simulink model "slmips"  (R2015a)
settings: Solver=FixedStepDiscrete  StartTime=0.0  StopTime=20  FixedStep=1  RelTol=1e-3
libraries: simulink x43, hdlsllib x22
settings Model: PauseTimes=1  SnapshotInterval=1  LastModifiedBy=peselnikmg
settings DataIOCC: SaveOutput=off  SaveTime=off
settings OptimizationCC: BlockReduction=off  ConditionallyExecuteInputs=off  InlineParams=on  OptimizeModelRefInitCode=on  LifeSpan=1
settings DebuggingCC: AlgebraicLoopMsg=error
settings HardwareCC: ProdHWDeviceType=ASIC/FPGA->ASIC/FPGA  TargetLongLongMode=on  TargetIntDivRoundTo=Zero  TargetEndianess=LittleEndian  TargetHWDeviceType=MATLAB Host  ProdEqTarget=off
settings RTWCC: SystemTargetFile=ert.tlc  GenCodeOnly=on  TemplateMakefile=ert_default_tmf  Description=Embedded Coder  GenerateReport=on  IncludeHyperlinkInReport=on  LaunchReport=on  GenerateTraceInfo=on  GenerateTraceReport=on  GenerateTraceReportSl=on  GenerateTraceReportSf=on  GenerateTraceReportEml=on
settings CodeAppCC: IgnoreCustomStorageClasses=off
settings ERTTargetCC: ParMdlRefBuildCompliant=on  CompOptLevelCompliant=on  ConcurrentExecutionCompliant=on  ERTFirstTimeCompliant=on  SupportContinuousTime=off  SupportVariableSizeSignals=off  ModelStepFunctionPrototypeControlCompliant=on  CPPClassGenCompliant=on  InlinedParameterPlacement=Hierarchical  ERTCustomFileTemplate=example_file_process.tlc

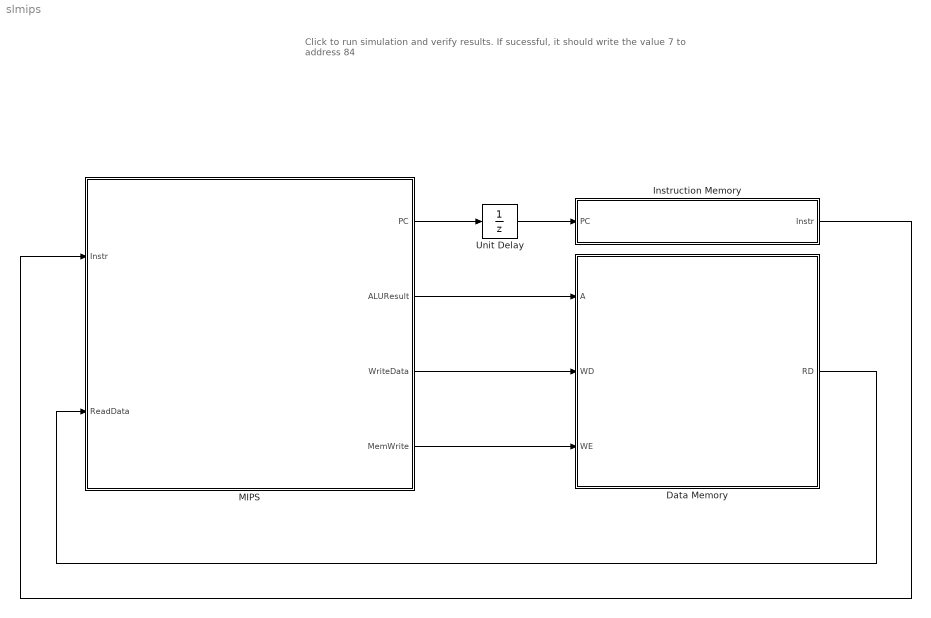
== system slmips ==
  note: Click to run simulation and verify results.
      | If sucessful, it should write the value 7 to address 84
  Data Memory : Subsystem
  Instruction Memory : Subsystem
  MIPS : Subsystem
  Unit Delay : UnitDelay  SampleTime=-1
  wires:
  MIPS/1(PC) -> Unit Delay/1
  Data Memory/1(RD) -> MIPS/2(ReadData)
  Instruction Memory/1(Instr) -> MIPS/1(Instr)
  Unit Delay/1 -> Instruction Memory/1(PC)
  MIPS/2(ALUResult) -> Data Memory/1(A)
  MIPS/3(WriteData) -> Data Memory/2(WD)
  MIPS/4(MemWrite) -> Data Memory/3(WE)

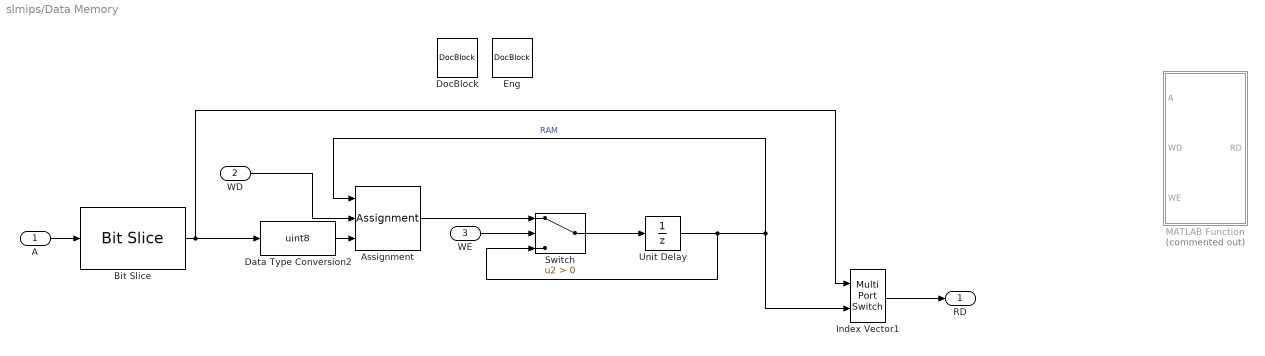
== system slmips/Data Memory ==
  A : Inport
  WD : Inport  Port=2
  WE : Inport  Port=3
  Assignment : Assignment  IndexMode=Zero-based  IndexOptions=Index vector (port)
  Bit Slice : hdlsllib/HDL Operations/Bit Slice  lidx=7  ridx=2
  Data Type Conversion2 : DataTypeConversion  OutDataTypeStr=uint8
  DocBlock : simulink/Model-Wide Utilities/DocBlock  DocumentType=Text
      content=|
      | Память данных имеет один порт чтения/записи. Если сигнал
      | разрешения записи WE равен единице, то данные со входа WD
      | записываются в ячейку памяти с адресом A по положительному фронту
      | тактового сигнала. Если же сигнал разрешения записи равен нулю,
      | то данные из ячейки с адресом A подаются на выход RD.
  Eng : simulink/Model-Wide Utilities/DocBlock  DocumentType=Text
      content=|
      | The data memory has a single read/write port. If the write enable,
      | WE, is 1, it writes data WD into address A on the rising edge of the clock.
      | If the write enable is 0, it reads address A onto RD.
  Index Vector1 : MultiPortSwitch  DataPortOrder=Zero-based contiguous  Inputs=1  zeroidx=on
  MATLAB Function : MATLAB Function  Commented=on  TreatAsAtomicUnit=on
  Switch : Switch  Criteria=u2 > Threshold
  Unit Delay : UnitDelay  InitialCondition=zeros(64,1)  SampleTime=-1
  RD : Outport  OutDataTypeStr=fixdt(0,32,0)
  wires:
  Unit Delay/1 -> Index Vector1/2, Assignment/1, Switch/3  "RAM"
  WE/1 -> Switch/2
  WD/1 -> Assignment/2
  Assignment/1 -> Switch/1
  Switch/1 -> Unit Delay/1
  Data Type Conversion2/1 -> Assignment/3
  Index Vector1/1 -> RD/1
  A/1 -> Bit Slice/1
  Bit Slice/1 -> Index Vector1/1, Data Type Conversion2/1

== system slmips/Instruction Memory ==
  PC : Inport
  DocBlock : simulink/Model-Wide Utilities/DocBlock  DocumentType=Text
      content=|
      | Память команд имеет один порт чтения. На адресный вход A подается
      | 32-битный адрес команды, после чего на выходе RD появляется
      | 32-битное число (т.е. команда), прочитанное из памяти по этому адресу.
  Eng : simulink/Model-Wide Utilities/DocBlock  DocumentType=Text
      content=|
      | The instruction memory has a single read port.1 It takes a 32-bit
      | instruction address input, A, and reads the 32-bit data (i.e., instruction)
      | from that address onto the read data output, RD.
  MATLAB Function : MATLAB Function  TreatAsAtomicUnit=on
  Instr : Outport  OutDataTypeStr=fixdt(0,32,0)
  wires:
  PC/1 -> MATLAB Function/1(PC)
  MATLAB Function/1(Instr) -> Instr/1  "Instr"

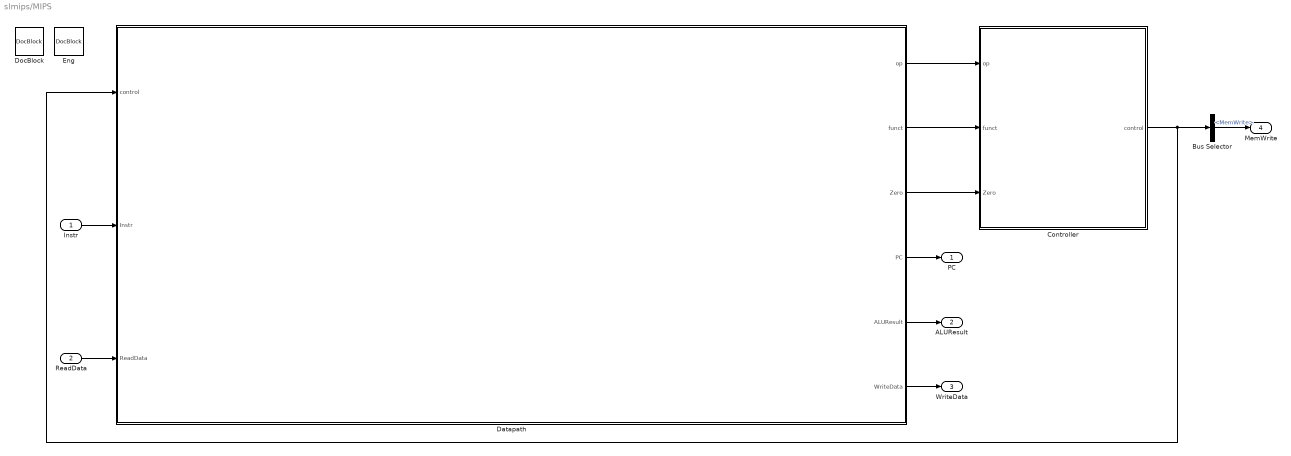
== system slmips/MIPS ==
  Instr : Inport
  ReadData : Inport  Port=2
  Bus Selector : BusSelector  OutputSignals=MemWrite
  Controller : Subsystem
  Datapath : Subsystem
  DocBlock : simulink/Model-Wide Utilities/DocBlock  DocumentType=Text
      content=|
      | Однотактовый процессор MIPS.
  Eng : simulink/Model-Wide Utilities/DocBlock  DocumentType=Text
      content=|
      | Single-cycle MIPS processor.
  PC : Outport
  ALUResult : Outport  Port=2
  WriteData : Outport  Port=3
  MemWrite : Outport  Port=4
  wires:
  Datapath/2(funct) -> Controller/2(funct)
  Datapath/1(op) -> Controller/1(op)
  Datapath/3(Zero) -> Controller/3(Zero)
  Datapath/4(PC) -> PC/1
  Instr/1 -> Datapath/2(Instr)
  ReadData/1 -> Datapath/3(ReadData)
  Datapath/6(WriteData) -> WriteData/1
  Datapath/5(ALUResult) -> ALUResult/1
  Bus Selector/1 -> MemWrite/1  "<MemWrite>"
  Controller/1(control) -> Datapath/1(control), Bus Selector/1

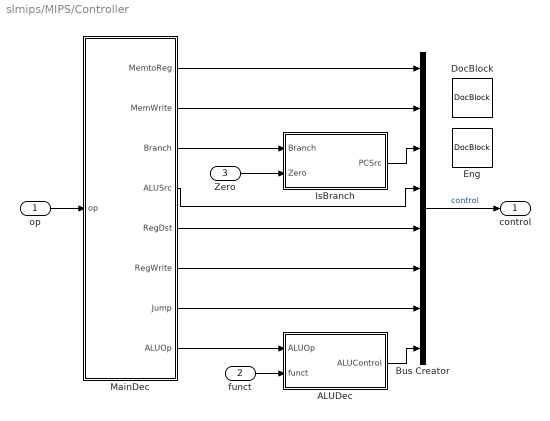
== system slmips/MIPS/Controller ==
  op : Inport
  funct : Inport  Port=2
  Zero : Inport  Port=3
  ALUDec : Subsystem
  Bus Creator : BusCreator  Inputs=8
  DocBlock : simulink/Model-Wide Utilities/DocBlock  DocumentType=Text
      content=|
      | Устройство управления формирует управляющие сигналы на основе
      | полей opcode и funct, присутствующих в каждой команде (Instr31:26 и
      | Instr5:0 соответственно).
  Eng : simulink/Model-Wide Utilities/DocBlock  DocumentType=Text
      content=|
      | The control unit computes the control signals based on the opcode and
      | funct fields of the instruction, Instr31:26 and Instr5:0.
  IsBranch : Subsystem
  MainDec : Subsystem
  control : Outport
  wires:
  Bus Creator/1 -> control/1  "control"
  MainDec/8(ALUOp) -> ALUDec/1(ALUOp)
  MainDec/3(Branch) -> IsBranch/1(Branch)
  op/1 -> MainDec/1(op)
  funct/1 -> ALUDec/2(funct)
  Zero/1 -> IsBranch/2(Zero)
  MainDec/1(MemtoReg) -> Bus Creator/1
  MainDec/2(MemWrite) -> Bus Creator/2
  IsBranch/1(PCSrc) -> Bus Creator/3
  MainDec/4(ALUSrc) -> Bus Creator/4
  MainDec/5(RegDst) -> Bus Creator/5
  MainDec/6(RegWrite) -> Bus Creator/6
  MainDec/7(Jump) -> Bus Creator/7
  ALUDec/1(ALUControl) -> Bus Creator/8

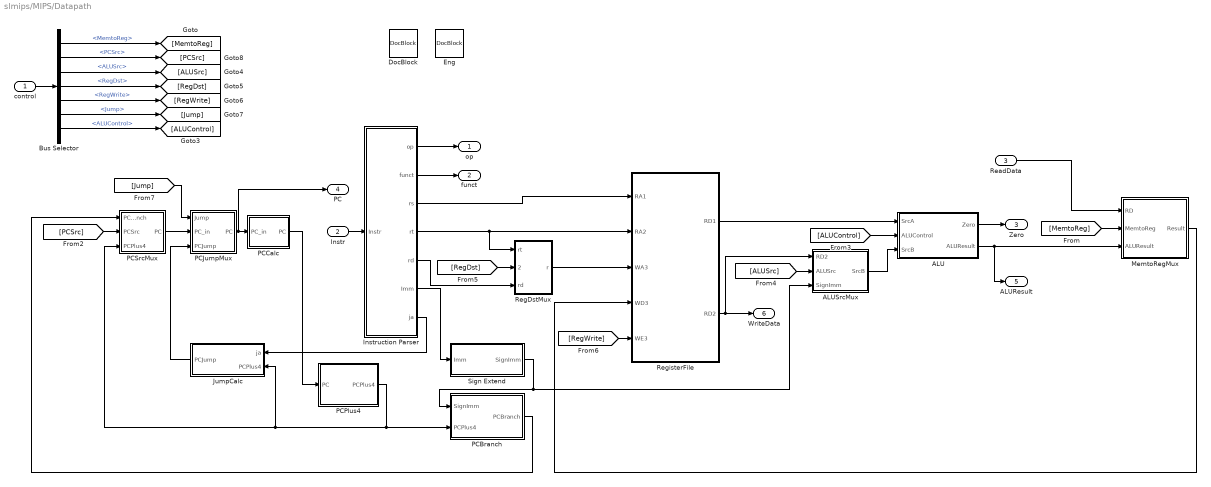
== system slmips/MIPS/Datapath ==
  control : Inport
  Instr : Inport  Port=2
  ReadData : Inport  Port=3
  ALU : Subsystem
  ALUSrcMux : Subsystem
  Bus Selector : BusSelector  OutputSignals=MemtoReg,PCSrc,ALUSrc,RegDst,RegWrite,Jump,ALUControl
  DocBlock : simulink/Model-Wide Utilities/DocBlock  DocumentType=Text
      content=|
      | Тракт данных однотактового процессора MIPS.
  Eng : simulink/Model-Wide Utilities/DocBlock  DocumentType=Text
      content=|
      | Datapath of a single-cycle MIPS processor.
  Instruction Parser : Subsystem
  JumpCalc : Subsystem
  MemtoRegMux : Subsystem
  PCBranch : Subsystem
  PCCalc : Subsystem
  PCJumpMux : Subsystem
  PCPlus4 : Subsystem
  PCSrcMux : Subsystem
  RegDstMux : Subsystem
  RegisterFile : Subsystem
  Sign Extend : Subsystem
  op : Outport
  funct : Outport  Port=2
  Zero : Outport  Port=3
  PC : Outport  Port=4
  ALUResult : Outport  Port=5
  WriteData : Outport  Port=6
  wires:
  Instruction Parser/4(rt) -> RegisterFile/2(RA2), RegDstMux/1(rt)
  [RegWrite] -> RegisterFile/5(WE3)
  Instruction Parser/3(rs) -> RegisterFile/1(RA1)
  ALUSrcMux/1(SrcB) -> ALU/3(SrcB)
  PCCalc/1(PC) -> PCPlus4/1(PC)
  [ALUSrc] -> ALUSrcMux/2(ALUSrc)
  RegisterFile/2(RD2) -> ALUSrcMux/1(RD2), WriteData/1
  [RegDst] -> RegDstMux/2(RegDst)
  [ALUControl] -> ALU/2(ALUControl)
  RegisterFile/1(RD1) -> ALU/1(SrcA)
  Sign Extend/1(SignImm) -> ALUSrcMux/3(SignImm), PCBranch/1(SignImm)
  RegDstMux/1(r) -> RegisterFile/3(WA3)
  [MemtoReg] -> MemtoRegMux/2(MemtoReg)
  Instr/1 -> Instruction Parser/1(Instr)
  Instruction Parser/2(funct) -> funct/1
  Instruction Parser/5(rd) -> RegDstMux/3(rd)
  Instruction Parser/6(Imm) -> Sign Extend/1(Imm)
  PCPlus4/1(PCPlus4) -> JumpCalc/2(PCPlus4), PCSrcMux/3(PCPlus4), PCBranch/2(PCPlus4)
  ALU/1(Zero) -> Zero/1
  PCBranch/1(PCBranch) -> PCSrcMux/1(PCBranch)
  Instruction Parser/1(op) -> op/1
  PCJumpMux/1(PC) -> PC/1, PCCalc/1(PC_in)
  [Jump] -> PCJumpMux/1(Jump)
  PCSrcMux/1(PC) -> PCJumpMux/2(PC_in)
  Instruction Parser/7(ja) -> JumpCalc/1(ja)
  JumpCalc/1(PCJump) -> PCJumpMux/3(PCJump)
  [PCSrc] -> PCSrcMux/2(PCSrc)
  control/1 -> Bus Selector/1
  Bus Selector/1 -> [MemtoReg]  "<MemtoReg>"
  Bus Selector/2 -> [PCSrc]  "<PCSrc>"
  Bus Selector/3 -> [ALUSrc]  "<ALUSrc>"
  Bus Selector/4 -> [RegDst]  "<RegDst>"
  Bus Selector/5 -> [RegWrite]  "<RegWrite>"
  Bus Selector/6 -> [Jump]  "<Jump>"
  Bus Selector/7 -> [ALUControl]  "<ALUControl>"
  ALU/2(ALUResult) -> MemtoRegMux/3(ALUResult), ALUResult/1
  ReadData/1 -> MemtoRegMux/1(RD)
  MemtoRegMux/1(Result) -> RegisterFile/4(WD3)

== system slmips/MIPS/Controller/ALUDec ==
  note: ALUOp
      | funct
      | ALUControl
      |
      | 00
      | X
      | 010 (addition)
      |
      | X1
      | X
      | 110 (subtraction)
      |
      | 1X
      | 100000
      | 010 (add)
      |
      | 1X
      | 100010
      | 110 (sub)
      |
      | 1X
      | 100100
      | 000 (and)
      |
      | 1X
      | 100101
      | 001 (or)
      |
      | 1X
      | 101010
      | 111 (slt)
  ALUOp : Inport
  funct : Inport  Port=2
  DocBlock : simulink/Model-Wide Utilities/DocBlock  DocumentType=Text
      content=|
      | Когда сигнал ALUOp равен 00 или 01, АЛУ должно складывать или
      | вычитать соответственно. Когда он равен 10, то значение ALUControl
      | должно определяться полем funct.
  Eng : simulink/Model-Wide Utilities/DocBlock  DocumentType=Text
      content=|
      | When ALUOp is 00 or 01,
      | the ALU should add or subtract, respectively. When ALUOp is 10, the
      | decoder examines the funct field to determine the ALUControl.
  MATLAB Function : MATLAB Function  TreatAsAtomicUnit=on
  ALUControl : Outport  OutDataTypeStr=fixdt(0,3,0)
  wires:
  ALUOp/1 -> MATLAB Function/1(ALUOp)
  funct/1 -> MATLAB Function/2(funct)
  MATLAB Function/1(ALUControl) -> ALUControl/1  "ALUControl"

== system slmips/MIPS/Controller/IsBranch ==
  Branch : Inport
  Zero : Inport  Port=2
  DocBlock : simulink/Model-Wide Utilities/DocBlock  DocumentType=Text
      content=|
      | Два регистра
      | сравниваются путем вычитания одного из другого в АЛУ. Если
      | ALUResult равен нулю, о чем сигнализирует флаг нуля, то регистры
      | равны. PCBranch
      | используется тогда, когда выполняется команда условного перехода и
      | установлен флаг нуля. Таким образом, сигнал Branch равен единице
      | для команды beq и нулю для прочих команд.
  Eng : simulink/Model-Wide Utilities/DocBlock  DocumentType=Text
      content=|
      | The two registers are compared by computing SrcA – SrcB using the
      | ALU. If ALUResult is 0, as indicated by the Zero flag from the ALU,
      | the registers are equal. We add a multiplexer to choose PC′ from either
      | PCPlus4 or PCBranch. PCBranch is selected if the instruction is a branch
      | and the Zero flag is asserted. Hence, Branch is 1 for beq and 0 for other
      | instructions.
  Logical Operator : Logic  AllPortsSameDT=off  OutDataTypeStr=fixdt(0,1,0)
  PCSrc : Outport
  wires:
  Zero/1 -> Logical Operator/2
  Logical Operator/1 -> PCSrc/1  "PCSrc"
  Branch/1 -> Logical Operator/1

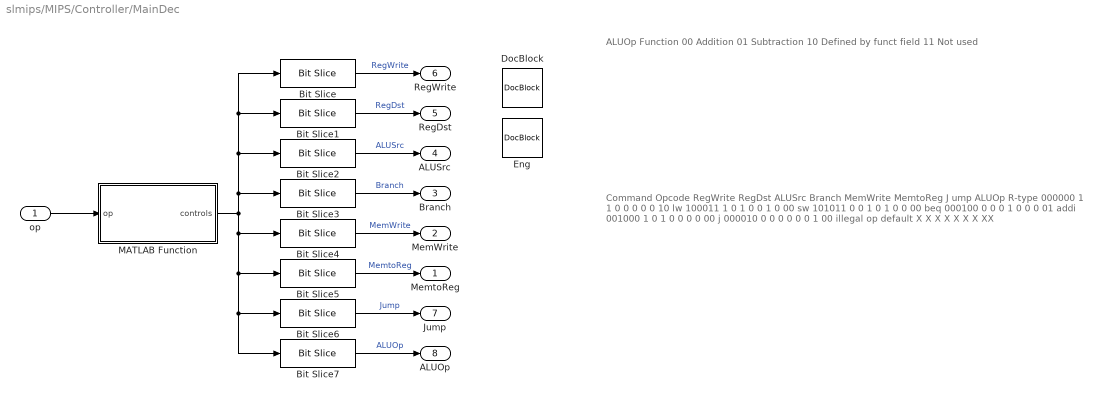
== system slmips/MIPS/Controller/MainDec ==
  note: Command
      | Opcode
      | RegWrite
      | RegDst
      | ALUSrc
      | Branch
      | MemWrite
      | MemtoReg
      | J ump
      | ALUOp
      |
      | R-type
      | 000000
      | 1
      | 1
      | 0
      | 0
      | 0
      | 0
      | 0
      | 10
      |
      | lw
      | 100011
      | 1
      | 0
      | 1
      | 0
      | 0
      | 1
      | 0
      | 00
      |
      | sw
      | 101011
      | 0
      | 0
      | 1
      | 0
      | 1
      | 0
      | 0
      | 00
      |
      | beq
      | 000100
      | 0
      | 0
      | 0
      | 1
      | 0
      | 0
      | 0
      | 01
      |
      | addi
      | 001000
      | 1
      | 0
      | 1
      | 0
      | 0
      | 0
      | 0
      | 00
      |
      | j
      | 000010
      | 0
      | 0
      | 0
      | 0
      | 0
      | 0
      | 1
      | 00
      |
      | illegal op
      | default
      | X
      | X
      | X
      | X
      | X
      | X
      | X
      | XX
  note: ALUOp
      | Function
      |
      | 00
      | Addition
      |
      | 01
      | Subtraction
      |
      | 10
      | Defined by funct field
      |
      | 11
      | Not used
  op : Inport
  Bit Slice : hdlsllib/HDL Operations/Bit Slice  lidx=8  ridx=8
  Bit Slice1 : hdlsllib/HDL Operations/Bit Slice  lidx=7  ridx=7
  Bit Slice2 : hdlsllib/HDL Operations/Bit Slice  lidx=6  ridx=6
  Bit Slice3 : hdlsllib/HDL Operations/Bit Slice  lidx=5  ridx=5
  Bit Slice4 : hdlsllib/HDL Operations/Bit Slice  lidx=4  ridx=4
  Bit Slice5 : hdlsllib/HDL Operations/Bit Slice  lidx=3  ridx=3
  Bit Slice6 : hdlsllib/HDL Operations/Bit Slice  lidx=2  ridx=2
  Bit Slice7 : hdlsllib/HDL Operations/Bit Slice  lidx=1  ridx=0
  DocBlock : simulink/Model-Wide Utilities/DocBlock  DocumentType=Text
      content=|
      | Основной дешифратор вычисляет значение большинства выходов на
      | основе поля opcode. Он также формирует двухбитный сигнал ALUOp.
      | Дешифратор АЛУ (ALU decoder) использует ALUOp совместно с полем
      | funct для вычисления состояния ALUControl. Расшифровка значений
      | сигнала ALUOp приведена в Таблице.
  Eng : simulink/Model-Wide Utilities/DocBlock  DocumentType=Text
      content=|
      | The main decoder
      | computes most of the outputs from the opcode. It also determines a 2-bit
      | ALUOp signal. The ALU decoder uses this ALUOp signal in conjunction
      | with the funct field to compute ALUControl. The meaning of the
      | ALUOp signal is given in Table.
  MATLAB Function : MATLAB Function  TreatAsAtomicUnit=on
  MemtoReg : Outport  OutDataTypeStr=fixdt(0,1,0)
  MemWrite : Outport  Port=2  OutDataTypeStr=fixdt(0,1,0)
  Branch : Outport  Port=3  OutDataTypeStr=fixdt(0,1,0)
  ALUSrc : Outport  Port=4  OutDataTypeStr=fixdt(0,1,0)
  RegDst : Outport  Port=5  OutDataTypeStr=fixdt(0,1,0)
  RegWrite : Outport  Port=6  OutDataTypeStr=fixdt(0,1,0)
  Jump : Outport  Port=7  OutDataTypeStr=fixdt(0,1,0)
  ALUOp : Outport  Port=8  OutDataTypeStr=fixdt(0,2,0)
  wires:
  op/1 -> MATLAB Function/1(op)
  MATLAB Function/1(controls) -> Bit Slice7/1, Bit Slice6/1, Bit Slice5/1, Bit Slice4/1, Bit Slice3/1, Bit Slice2/1, Bit Slice1/1, Bit Slice/1
  Bit Slice/1 -> RegWrite/1  "RegWrite"
  Bit Slice1/1 -> RegDst/1  "RegDst"
  Bit Slice2/1 -> ALUSrc/1  "ALUSrc"
  Bit Slice3/1 -> Branch/1  "Branch"
  Bit Slice4/1 -> MemWrite/1  "MemWrite"
  Bit Slice5/1 -> MemtoReg/1  "MemtoReg"
  Bit Slice6/1 -> Jump/1  "Jump"
  Bit Slice7/1 -> ALUOp/1  "ALUOp"

== system slmips/MIPS/Datapath/ALU ==
  note: ALUControl
      |
      | 010 (add)
      |
      | 110 (sub)
      |
      | 000 (and)
      |
      | 001 (or)
      |
      | 111 (slt)
  SrcA : Inport
  ALUControl : Inport  Port=2
  SrcB : Inport  Port=3
  DocBlock : simulink/Model-Wide Utilities/DocBlock  DocumentType=Text
      content=|
      | АЛУ получает на входы два операнда, SrcA и SrcB.
      | Трехбитный управляющий сигнал ALUControl
      | говорит АЛУ, какую операцию надо выполнить. На выходе из АЛУ
      | получается 32-битный результат ALUResult и флаг нуля (Zero flag),
      | который устанавливается в единицу, если ALUResult равен нулю.
  Eng : simulink/Model-Wide Utilities/DocBlock  DocumentType=Text
      content=|
      | The ALU receives two operands, SrcA and SrcB. SrcA
      | comes from the register file, and SrcB comes from the sign-extended
      | immediate. The 3-bit ALUControl signal specifies the operation. The
      | ALU generates a 32-bit ALUResult and a Zero flag, that indicates
      | whether ALUResult == 0.
  MATLAB Function : MATLAB Function  TreatAsAtomicUnit=on
  Zero : Outport  OutDataTypeStr=fixdt(0,1,0)
  ALUResult : Outport  Port=2  OutDataTypeStr=fixdt(0,32,0)
  wires:
  ALUControl/1 -> MATLAB Function/1(ALUControl)
  SrcA/1 -> MATLAB Function/2(SrcA)
  SrcB/1 -> MATLAB Function/3(SrcB)
  MATLAB Function/1(ALUResult) -> ALUResult/1
  MATLAB Function/2(Zero) -> Zero/1

== system slmips/MIPS/Datapath/ALUSrcMux ==
  RD2 : Inport
  ALUSrc : Inport  Port=2
  SignImm : Inport  Port=3
  ALUSrcMux : Switch  Criteria=u2 > Threshold
  DocBlock : simulink/Model-Wide Utilities/DocBlock  DocumentType=Text
      content=|
      | Нам пришлось добавить мультиплексор, чтобы была возможность
      | подать на вход АЛУ или SignImm, или выход RD2 регистрового файла.
      | Мультиплексор управляется новым сигналом ALUSrc.
      | ALUSrc равен нулю для команд типа R – в этом случае на вход АЛУ подается
      | значение из регистрового файла. Для команд lw и sw ALUSrc равен
      | единице, и на вход АЛУ подается SignImm.
  Eng : simulink/Model-Wide Utilities/DocBlock  DocumentType=Text
      content=|
      | The multiplexer to choose SrcB from either the register file RD2 port
      | or SignImm.
      | The multiplexer is controlled by a new signal, ALUSrc. ALUSrc is 0
      | for R-type instructions to choose SrcB from the register file; it is 1 for
      | lw and sw to choose SignImm. This principle of enhancing the datapath’s
      | capabilities by adding a multiplexer to choose inputs from several possibilities
      | is extremely useful. Indeed, we will apply it twice more to complete
      | the handling of R-type instructions.
  SrcB : Outport
  wires:
  ALUSrc/1 -> ALUSrcMux/2
  ALUSrcMux/1 -> SrcB/1
  SignImm/1 -> ALUSrcMux/1
  RD2/1 -> ALUSrcMux/3

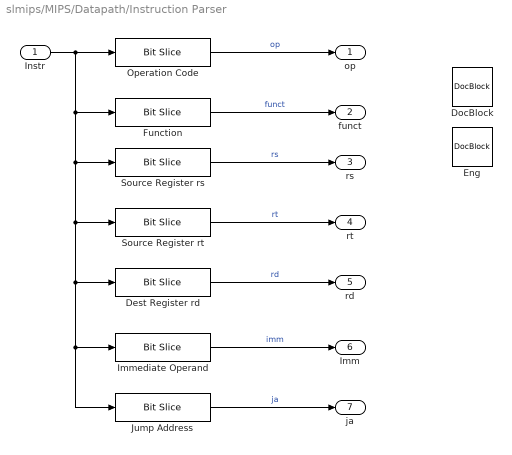
== system slmips/MIPS/Datapath/Instruction Parser ==
  Instr : Inport
  Dest Register rd : hdlsllib/HDL Operations/Bit Slice  lidx=15  ridx=11
  DocBlock : simulink/Model-Wide Utilities/DocBlock  DocumentType=Text
      content=|
      | Refer to MIPS machine code description.
  Eng : simulink/Model-Wide Utilities/DocBlock  DocumentType=Text
      content=|
      | Refer to MIPS machine code description.
  Function : hdlsllib/HDL Operations/Bit Slice  lidx=5  ridx=0
  Immediate Operand : hdlsllib/HDL Operations/Bit Slice  lidx=15  ridx=0
  Jump Address : hdlsllib/HDL Operations/Bit Slice  lidx=25  ridx=0
  Operation Code : hdlsllib/HDL Operations/Bit Slice  lidx=31  ridx=26
  Source Register rs : hdlsllib/HDL Operations/Bit Slice  lidx=25  ridx=21
  Source Register rt : hdlsllib/HDL Operations/Bit Slice  lidx=20  ridx=16
  op : Outport
  funct : Outport  Port=2
  rs : Outport  Port=3
  rt : Outport  Port=4
  rd : Outport  Port=5
  Imm : Outport  Port=6
  ja : Outport  Port=7
  wires:
  Source Register rs/1 -> rs/1  "rs"
  Immediate Operand/1 -> Imm/1  "imm"
  Source Register rt/1 -> rt/1  "rt"
  Dest Register rd/1 -> rd/1  "rd"
  Instr/1 -> Operation Code/1, Function/1, Jump Address/1, Immediate Operand/1, Dest Register rd/1, Source Register rt/1, Source Register rs/1
  Operation Code/1 -> op/1  "op"
  Function/1 -> funct/1  "funct"
  Jump Address/1 -> ja/1  "ja"

== system slmips/MIPS/Datapath/JumpCalc ==
  note: Do we need this? From diagram on p. 960, seems yes.. But logically - no!
  ja : Inport
  PCPlus4 : Inport  Port=2
  Bit Concat : hdlsllib/HDL Operations/Bit Concat  numInputs=3
  Bit Shift : hdlsllib/HDL Operations/Bit Shift  Commented=through  mode=Shift Left Logical  N=2
  Constant : Constant  Value=0  OutDataTypeStr=fixdt(0,2,0)
  DocBlock : simulink/Model-Wide Utilities/DocBlock  DocumentType=Text
      content=|
      | Команда безусловного перехода j записывает новое значение в счетчик команд.
      | Два младших бита нового значения всегда равны нулю, потому что длина любой
      | команды равна четырем байтам, следовательно, ее адрес всегда кратен
      | четырем. Следующие 26 бит процессор возьмет из поля адреса перехода (jump
      | address field) Instr25:0. Четыре оставшихся старших бита будут равны четырем
      | старшим битам предыдущего значения счетчика команд.
  Eng : simulink/Model-Wide Utilities/DocBlock  DocumentType=Text
      content=|
      | The jump instruction, j, writes a new value into the PC. The two least significant
      | bits of the PC are always 0, because the PC is word aligned (i.e., always a multiple
      | of 4). The next 26 bits are taken from the jump address field in Instr25:0. The
      | upper four bits are taken from the old value of the PC.
  Operation Code : hdlsllib/HDL Operations/Bit Slice  lidx=31  ridx=28
  PCJump : Outport
  wires:
  Bit Concat/1 -> PCJump/1
  PCPlus4/1 -> Operation Code/1
  ja/1 -> Bit Concat/2
  Operation Code/1 -> Bit Concat/1
  Constant/1 -> Bit Concat/3

== system slmips/MIPS/Datapath/MemtoRegMux ==
  RD : Inport
  MemtoReg : Inport  Port=2
  ALUResult : Inport  Port=3
  DocBlock : simulink/Model-Wide Utilities/DocBlock  DocumentType=Text
      content=|
      | Команды типа R должны записывать в
      | регистровый файл значение ALUResult. Чтобы выбирать между
      | ReadData и ALUResult, мы добавляем этот мультиплексор.
      | Этот мультиплексор управляется сигналом MemtoReg.
      | MemtoReg равен нулю для команд
      | типа R – в этом случае Result принимает значение ALUResult.
      | Для команды lw MemtoReg равен единице, а Result принимает
      | значение ReadData. Для команды sw значение MemtoReg не играет
      | никакой роли, так как sw ничего в регистровый файл не пишет.
  Eng : simulink/Model-Wide Utilities/DocBlock  DocumentType=Text
      content=|
      | R-type instructions write the ALUResult to the register
      | file. Therefore, we add this multiplexer to choose between ReadData
      | and ALUResult. We call its output Result. This multiplexer is
      | controlled by signal MemtoReg. MemtoReg is 0 for R-type
      | instructions to choose Result from the ALUResult; it is 1 for lw to choose
      | ReadData. We don’t care about the value of MemtoReg for sw, because
      | sw does not write to the register file.
  MemtoRegMux : Switch  Criteria=u2 > Threshold
  Result : Outport
  wires:
  MemtoReg/1 -> MemtoRegMux/2
  MemtoRegMux/1 -> Result/1
  RD/1 -> MemtoRegMux/1
  ALUResult/1 -> MemtoRegMux/3

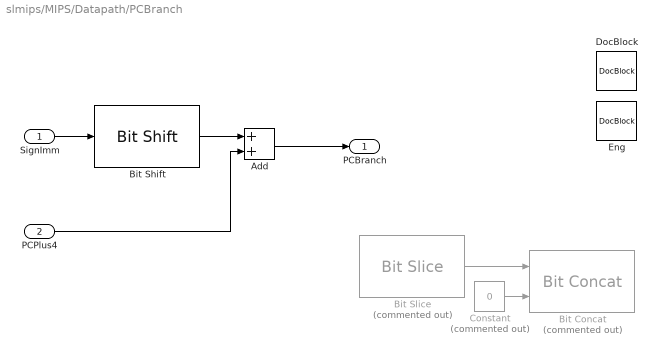
== system slmips/MIPS/Datapath/PCBranch ==
  SignImm : Inport
  PCPlus4 : Inport  Port=2
  Add : Sum  AccumDataTypeStr=fixdt(0,32,0)  OutDataTypeStr=fixdt(0,32,0)
  Bit Concat : hdlsllib/HDL Operations/Bit Concat  Commented=on  numInputs=2
  Bit Shift : hdlsllib/HDL Operations/Bit Shift  mode=Shift Left Logical  N=2
  Bit Slice : hdlsllib/HDL Operations/Bit Slice  Commented=on  lidx=29  ridx=0
  Constant : Constant  Commented=on  Value=0  OutDataTypeStr=fixdt(0,2,0)
  DocBlock : simulink/Model-Wide Utilities/DocBlock  DocumentType=Text
      content=|
      | Смещение указывает, сколько команд нужно перепрыгнуть, прежде чем
      | продолжить выполнение программы. Таким образом, над значением
      | непосредственного операнда надо выполнить операцию знакового
      | расширения, поле чего умножить его на четыре, чтобы получить новое
      | значение счетчика команд: PC_in = PC + 4 + SignImm * 4.
      | Новое значение счетчика команд на случай выполненного
      | условного перехода (PCBranch) вычисляется путем сдвига SignImm
      | влево на два разряда и последующего сложения с PCPlus4.
  Eng : simulink/Model-Wide Utilities/DocBlock  DocumentType=Text
      content=|
      | The offset
      | indicates the number of instructions to branch past. Hence, the immediate
      | must be sign-extended and multiplied by 4 to get the new program counter
      | value: PC′ = PC + 4 + SignImm × 4.
      | The next PC value
      | for a taken branch, PCBranch, is computed by shifting SignImm left
      | by 2 bits, then adding it to PCPlus4.
  PCBranch : Outport
  wires:
  SignImm/1 -> Bit Shift/1
  PCPlus4/1 -> Add/2
  Bit Shift/1 -> Add/1
  Add/1 -> PCBranch/1
  Bit Slice/1 -> Bit Concat/1
  Constant/1 -> Bit Concat/2

== system slmips/MIPS/Datapath/PCCalc ==
  PC_in : Inport
  DocBlock : simulink/Model-Wide Utilities/DocBlock  DocumentType=Text
      content=|
      | Счетчик команд – это обычный 32-битный регистр. Его выход (PC)
      | содержит адрес текущей команды. Его вход (PC_in) содержит адрес
      | следующей команды.
  Eng : simulink/Model-Wide Utilities/DocBlock  DocumentType=Text
      content=|
      | The program counter is an ordinary 32-bit register. Its output, PC,
      | points to the current instruction. Its input, PC′, indicates the address of
      | the next instruction.
  PC Start : UnitDelay  Description=Начальное значение счетчика команд.  SampleTime=-1
  PC : Outport  OutDataTypeStr=fixdt(0,32,0)
  wires:
  PC_in/1 -> PC Start/1
  PC Start/1 -> PC/1  "PC"

== system slmips/MIPS/Datapath/PCJumpMux ==
  Jump : Inport
  PC_in : Inport  Port=2
  PCJump : Inport  Port=3
  DocBlock : simulink/Model-Wide Utilities/DocBlock  DocumentType=Text
      content=|
      | Команда безусловного перехода j записывает новое значение в счетчик команд.
      | Два младших бита нового значения всегда равны нулю, потому что длина любой
      | команды равна четырем байтам, следовательно, ее адрес всегда кратен
      | четырем. Следующие 26 бит процессор возьмет из поля адреса перехода (jump
      | address field) Instr25:0. Четыре оставшихся старших бита будут равны четырем
      | старшим битам предыдущего значения счетчика команд.
  Eng : simulink/Model-Wide Utilities/DocBlock  DocumentType=Text
      content=|
      | The jump instruction, j, writes a new value into the PC. The two least significant
      | bits of the PC are always 0, because the PC is word aligned (i.e., always a multiple
      | of 4). The next 26 bits are taken from the jump address field in Instr25:0. The
      | upper four bits are taken from the old value of the PC.
  PCJumpMux : Switch  Criteria=u2 > Threshold
  PC : Outport
  wires:
  PCJumpMux/1 -> PC/1
  Jump/1 -> PCJumpMux/2
  PCJump/1 -> PCJumpMux/1
  PC_in/1 -> PCJumpMux/3

== system slmips/MIPS/Datapath/PCPlus4 ==
  PC : Inport
  DocBlock : simulink/Model-Wide Utilities/DocBlock  DocumentType=Text
      content=|
      | Одновременно с выполнением команды процессор должен вычислить
      | адрес следующей команды, PC_in. Так как команды 32-битные, то есть
      | четырехбайтные, то адрес следующей команды равен PC + 4.
  Eng : simulink/Model-Wide Utilities/DocBlock  DocumentType=Text
      content=|
      | While the instruction is being executed, the processor must compute the
      | address of the next instruction, PC′. Because instructions are 32 bits =
      | 4 bytes, the next instruction is at PC + 4.
  PCInc : Bias  Bias=4
  PCPlus4 : Outport
  wires:
  PC/1 -> PCInc/1
  PCInc/1 -> PCPlus4/1

== system slmips/MIPS/Datapath/PCSrcMux ==
  PCBranch : Inport
  PCSrc : Inport  Port=2
  PCPlus4 : Inport  Port=3
  DocBlock : simulink/Model-Wide Utilities/DocBlock  DocumentType=Text
      content=|
      | Мультиплексор, чтобы выбрать, какое именно
      | значение присвоить PC_in – PCPlus4 или PCBranch. PCBranch
      | используется тогда, когда выполняется команда условного перехода и
      | установлен флаг нуля.
  Eng : simulink/Model-Wide Utilities/DocBlock  DocumentType=Text
      content=|
      | The multiplexer to choose PC′ from either
      | PCPlus4 or PCBranch. PCBranch is selected if the instruction is a branch
      | and the Zero flag is asserted.
  PCSrcMux : Switch  Criteria=u2 > Threshold
  PC : Outport
  wires:
  PCSrc/1 -> PCSrcMux/2
  PCPlus4/1 -> PCSrcMux/3
  PCSrcMux/1 -> PC/1
  PCBranch/1 -> PCSrcMux/1

== system slmips/MIPS/Datapath/RegDstMux ==
  rt : Inport
  RegDst : Inport  Port=2
  rd : Inport  Port=3
  DocBlock : simulink/Model-Wide Utilities/DocBlock  DocumentType=Text
      content=|
      | Этот мультиплексор
      | управляется сигналом RegDst. RegDst равен единице для команд
      | типа R – в этом случае выход принимает значение поля rd (Instr15:11).
      | Для команды lw RegDst равен нулю, а выход принимает значение
      | поля rt (Instr20:16). Для команды sw значение RegDst не играет никакой
      | роли, так как sw ничего в регистровый файл не пишет.
  Eng : simulink/Model-Wide Utilities/DocBlock  DocumentType=Text
      content=|
      | The multiplexer is controlled by RegDst. RegDst is 1 for R-type
      | instructions to choose WriteReg from the rd field, Instr15:11; it is 0 for
      | lw to choose the rt field, Instr20:16. We don’t care about the value of
      | RegDst for sw, because sw does not write to the register file.
  RegDstMux : Switch  Criteria=u2 > Threshold
  r : Outport
  wires:
  RegDst/1 -> RegDstMux/2
  RegDstMux/1 -> r/1
  rt/1 -> RegDstMux/3
  rd/1 -> RegDstMux/1

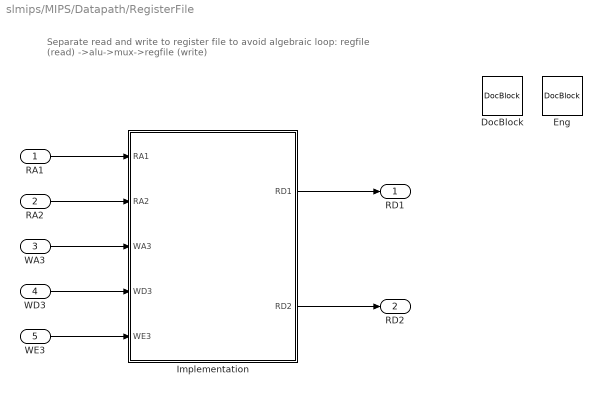
== system slmips/MIPS/Datapath/RegisterFile ==
  note: Separate read and write to register file to avoid algebraic loop:
      | regfile (read) ->alu->mux->regfile (write)
  RA1 : Inport
  RA2 : Inport  Port=2
  WA3 : Inport  Port=3
  WD3 : Inport  Port=4
  WE3 : Inport  Port=5
  DocBlock : simulink/Model-Wide Utilities/DocBlock  DocumentType=Text
      content=|
      | Регистровый файл, содержащий 32 элемента по 32 бита каждый, имеет
      | два порта чтения и один порт записи данных. Порты чтения имеют
      | пятибитные входы адреса A1 и A2, каждый из которых определяет один
      | из 2^5 = 32 регистров в качестве источника данных для команды. Каждый
      | из портов читает 32-битное значение из регистра и подает его на
      | выходы RD1 и RD2 соответственно. Порт записи получает пятибитный
      | адрес регистра на адресный вход A3, 32-битное число на вход данных
      | WD, сигнал разрешения записи WE3 и тактовый сигнал. Если сигнал
      | разрешения записи равен единице, то регистровый файл записывает
      | данные в указанный регистр по положительному фронту тактового
      | сигнала.
  Eng : simulink/Model-Wide Utilities/DocBlock  DocumentType=Text
      content=|
      | The 32-element × 32-bit register file has two read ports and one write
      | port. The read ports take 5-bit address inputs, A1 and A2, each specifying
      | one of 25 = 32 registers as source operands. They read the 32-bit register
      | values onto read data outputs RD1 and RD2, respectively. The write port
      | takes a 5-bit address input, A3; a 32-bit write data input, WD; a write
      | enable input, WE3; and a clock. If the write enable is 1, the register file
      | writes the data into the specified register on the rising edge of the clock.
  Implementation : Subsystem  Variant=on  OverrideUsingVariant=SL_impl_BB
  RD1 : Outport  OutDataTypeStr=fixdt(0,32,0)
  RD2 : Outport  Port=2  OutDataTypeStr=fixdt(0,32,0)
  wires:
  RA1/1 -> Implementation/1(RA1)
  RA2/1 -> Implementation/2(RA2)
  WA3/1 -> Implementation/3(WA3)
  WD3/1 -> Implementation/4(WD3)
  WE3/1 -> Implementation/5(WE3)
  Implementation/1(RD1) -> RD1/1
  Implementation/2(RD2) -> RD2/1

== system slmips/MIPS/Datapath/Sign Extend ==
  note: TODO: check if it works with jumping back. PCBranch must decrement in this case.
  Imm : Inport
  Data Type Conversion : DataTypeConversion  Commented=on  ConvertRealWorld=Stored Integer (SI)
  DocBlock : simulink/Model-Wide Utilities/DocBlock  DocumentType=Text
      content=|
      | Команде lw также требуется смещение (offset) – число, которое будет
      | прибавлено к базовому адресу. Смещение передается как
      | непосредственный операнд (immediate), то есть находится
      | непосредственно в поле Instr15:0, занимая младшие 16 бит. Так как
      | 16-битное число может быть как положительным, так и отрицательным,
      | то над ним должна быть выполнена операция знакового расширения до
      | 32 бит. Полученное 32-битное расширенное значение называется SignImm.
      | Знаковое расширение заключается в том, что знаковый бит (он же
      | старший бит) расширяемого числа просто копируется во все старшие
      | биты расширенного числа, а именно SignImm15:0 = Instr15:0 и
      | SignImm31:16 = Instr15.
  Eng : simulink/Model-Wide Utilities/DocBlock  DocumentType=Text
      content=|
      | The lw instruction also requires an offset. The offset is stored in the
      | immediate field of the instruction, Instr15:0. Because the 16-bit immediate
      | might be either positive or negative, it must be sign-extended to 32 bits.
      | The 32-bit sign-extended value is called SignImm.
      | Sign extension simply copies the sign bit
      | (most significant bit) of a short input into all of the upper bits of the
      | longer output. Specifically, SignImm15:0 = Instr15:0 and SignImm31:16 =
      | Instr15.
  MATLAB Function : MATLAB Function  TreatAsAtomicUnit=on
  SignImm : Outport  OutDataTypeStr=fixdt(0,32,0)
  wires:
  Imm/1 -> MATLAB Function/1(a)
  MATLAB Function/1(y) -> SignImm/1

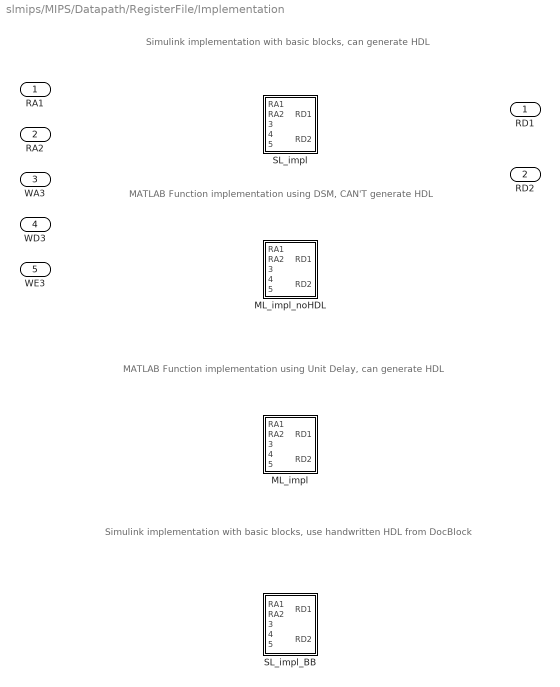
== system slmips/MIPS/Datapath/RegisterFile/Implementation ==
  note: MATLAB Function implementation using DSM, CAN'T generate HDL
  note: Simulink implementation with basic blocks, can generate HDL
  note: MATLAB Function implementation using Unit Delay, can generate HDL
  note: Simulink implementation with basic blocks, use handwritten HDL from DocBlock
  RA1 : Inport
  RA2 : Inport  Port=2
  WA3 : Inport  Port=3
  WD3 : Inport  Port=4
  WE3 : Inport  Port=5
  ML_impl : Subsystem  VariantControl=ML_impl
  ML_impl_noHDL : Subsystem  VariantControl=ML_impl_noHDL
  SL_impl : Subsystem  VariantControl=SL_impl
  SL_impl_BB : Subsystem  VariantControl=SL_impl_BB
  RD1 : Outport  OutDataTypeStr=fixdt(0,32,0)
  RD2 : Outport  Port=2  OutDataTypeStr=fixdt(0,32,0)

== system slmips/MIPS/Datapath/RegisterFile/Implementation/ML_impl ==
  RA1 : Inport
  RA2 : Inport  Port=2
  WA3 : Inport  Port=3
  WD3 : Inport  Port=4
  WE3 : Inport  Port=5
  Read : MATLAB Function  TreatAsAtomicUnit=on
  Unit Delay : UnitDelay  InitialCondition=zeros(32,1)  SampleTime=-1
  Write : MATLAB Function  TreatAsAtomicUnit=on
  RD1 : Outport  OutDataTypeStr=fixdt(0,32,0)
  RD2 : Outport  Port=2  OutDataTypeStr=fixdt(0,32,0)
  wires:
  WD3/1 -> Write/2(WD3)
  RA1/1 -> Read/1(RA1)
  RA2/1 -> Read/2(RA2)
  WA3/1 -> Write/1(WA3)
  WE3/1 -> Write/3(WE3)
  Read/2(RD2) -> RD2/1
  Read/1(RD1) -> RD1/1
  Write/1(regfile_wr) -> Unit Delay/1
  Unit Delay/1 -> Write/4(regfile), Read/3(regfile)

== system slmips/MIPS/Datapath/RegisterFile/Implementation/ML_impl_noHDL ==
  RA1 : Inport
  RA2 : Inport  Port=2
  WA3 : Inport  Port=3
  WD3 : Inport  Port=4
  WE3 : Inport  Port=5
  Data Store Memory : DataStoreMemory  DataStoreName=regfile  WriteAfterWriteMsg=warning  InitialValue=zeros(32,1)  OutDataTypeStr=fixdt(0,32,0)
  Read : MATLAB Function  TreatAsAtomicUnit=on
  Write : MATLAB Function  TreatAsAtomicUnit=on
  RD1 : Outport  OutDataTypeStr=fixdt(0,32,0)
  RD2 : Outport  Port=2  OutDataTypeStr=fixdt(0,32,0)
  wires:
  Read/1(RD1) -> RD1/1
  Read/2(RD2) -> RD2/1
  WE3/1 -> Write/3(WE3)
  WA3/1 -> Write/1(WA3)
  RA2/1 -> Read/2(RA2)
  RA1/1 -> Read/1(RA1)
  WD3/1 -> Write/2(WD3)

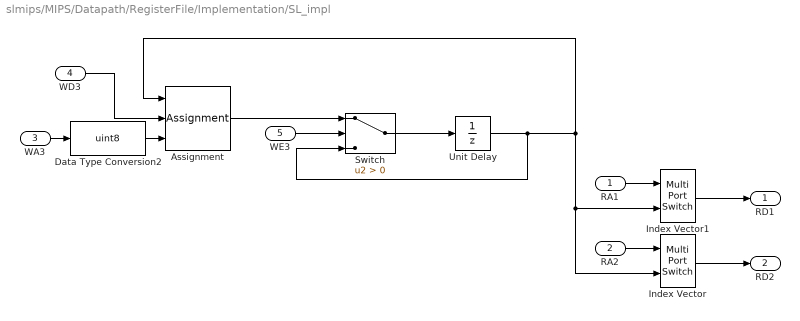
== system slmips/MIPS/Datapath/RegisterFile/Implementation/SL_impl ==
  RA1 : Inport
  RA2 : Inport  Port=2
  WA3 : Inport  Port=3
  WD3 : Inport  Port=4
  WE3 : Inport  Port=5
  Assignment : Assignment  IndexMode=Zero-based  IndexOptions=Index vector (port)
  Data Type Conversion2 : DataTypeConversion  OutDataTypeStr=uint8
  Index Vector : MultiPortSwitch  DataPortOrder=Zero-based contiguous  Inputs=1  zeroidx=on
  Index Vector1 : MultiPortSwitch  DataPortOrder=Zero-based contiguous  Inputs=1  zeroidx=on
  Switch : Switch  Criteria=u2 > Threshold
  Unit Delay : UnitDelay  InitialCondition=zeros(32,1)  SampleTime=-1
  RD1 : Outport  OutDataTypeStr=fixdt(0,32,0)
  RD2 : Outport  Port=2  OutDataTypeStr=fixdt(0,32,0)
  wires:
  Unit Delay/1 -> Index Vector1/2, Index Vector/2, Assignment/1, Switch/3
  Index Vector/1 -> RD2/1
  RA2/1 -> Index Vector/1
  WE3/1 -> Switch/2
  WA3/1 -> Data Type Conversion2/1
  WD3/1 -> Assignment/2
  Assignment/1 -> Switch/1
  Switch/1 -> Unit Delay/1
  Data Type Conversion2/1 -> Assignment/3
  RA1/1 -> Index Vector1/1
  Index Vector1/1 -> RD1/1

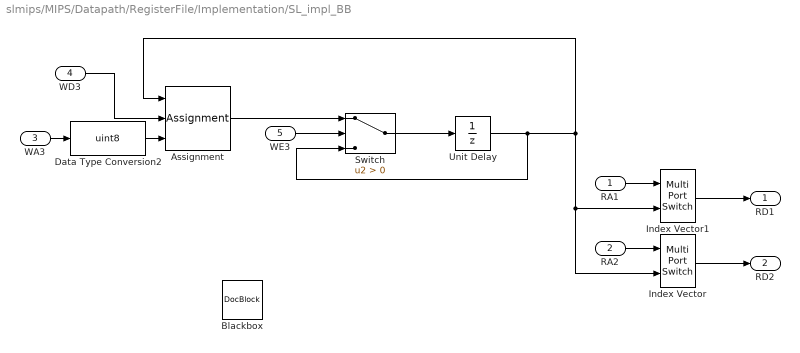
== system slmips/MIPS/Datapath/RegisterFile/Implementation/SL_impl_BB ==
  RA1 : Inport
  RA2 : Inport  Port=2
  WA3 : Inport  Port=3
  WD3 : Inport  Port=4
  WE3 : Inport  Port=5
  Assignment : Assignment  IndexMode=Zero-based  IndexOptions=Index vector (port)
  Blackbox : simulink/Model-Wide Utilities/DocBlock  DocumentType=Text
      content=|
      | module SL_impl_BB(
      |            clk,
      |            RA1,
      |            RA2,
      |            WA3,
      |            WD3,
      |            WE3,
      |            RD1,
      |            RD2
      |           );
      |
      | input   clk;
      | input   [4:0] RA1;  // ufix5
      | input   [4:0] RA2;  // ufix5
      | input   [4:0] WA3;  // ufix5
      | input   [31:0] WD3;  // uint32
      | input   WE3;  // ufix1
      | output  [31:0] RD1;  // uint32
      | output  [31:0] RD2;  // uint32
      |
      | reg [31:0] rf[31:0];
      |
      | always @(posedge clk)
      |     if (WE3) rf[WA3] <= WD3;
      |
      | assign RD1 = (RA1 != 0) ? rf[RA1] : 0;
      | assign RD2 = (RA2 != 0) ? rf[RA2] : 0;
      |
      | endmodule
  Data Type Conversion2 : DataTypeConversion  OutDataTypeStr=uint8
  Index Vector : MultiPortSwitch  DataPortOrder=Zero-based contiguous  Inputs=1  zeroidx=on
  Index Vector1 : MultiPortSwitch  DataPortOrder=Zero-based contiguous  Inputs=1  zeroidx=on
  Switch : Switch  Criteria=u2 > Threshold
  Unit Delay : UnitDelay  InitialCondition=zeros(32,1)  SampleTime=-1
  RD1 : Outport  OutDataTypeStr=fixdt(0,32,0)
  RD2 : Outport  Port=2  OutDataTypeStr=fixdt(0,32,0)
  wires:
  Unit Delay/1 -> Index Vector1/2, Index Vector/2, Assignment/1, Switch/3
  Index Vector/1 -> RD2/1
  RA2/1 -> Index Vector/1
  WE3/1 -> Switch/2
  WA3/1 -> Data Type Conversion2/1
  WD3/1 -> Assignment/2
  Assignment/1 -> Switch/1
  Switch/1 -> Unit Delay/1
  Data Type Conversion2/1 -> Assignment/3
  RA1/1 -> Index Vector1/1
  Index Vector1/1 -> RD1/1

== matlab function slmips/MIPS/Datapath/ALU/MATLAB Function ==
  settings: fimath=|
      | fimath(...
      | 'RoundMode', 'floor',...
      | 'OverflowMode', 'wrap',...
      | 'ProductMode', 'FullPrecision', 'ProductWordLength', 32,...
      | 'SumMode', 'FullPrecision', 'SumWordLength', 32,...
      | 'CastBeforeSum', true);
  data: ALUControl input fixdt(0,3,0); ALUResult output fixdt(0,32,0); SrcA input fixdt(0,32,0); SrcB input fixdt(0,32,0); Zero output fixdt(0,1,0)
function [ALUResult, Zero] = fcn(ALUControl, SrcA, SrcB)
%#codegen

ALUResult = fi(0,0,32,0);
Zero = fi(0,0,1,0);

switch ALUControl
    case bin2dec('010')
        %add
        ALUResult(:) = SrcA + SrcB;
    case bin2dec('110')
        %sub
        ALUResult(:) = SrcA - SrcB;
    case bin2dec('000')
        %and
        ALUResult(:) = bitand(SrcA, SrcB);
    case bin2dec('001')
        %or
        ALUResult(:) = bitor(SrcA, SrcB);
    case bin2dec('111')
        %slt
        if (SrcA < SrcB)
            ALUResult(:) = 1;
        else
            ALUResult(:) = 0;
        end
    otherwise
end

%slt
if (ALUResult == 0)
    Zero(:) = 1;
else
    Zero(:) = 0;
end

== matlab function slmips/MIPS/Datapath/Sign Extend/MATLAB Function ==
  data: a input fixdt(0,16,0); y output fixdt(0,32,0)
function y = fcn(a)
%#codegen

%Output is a signed value
y = bitconcat(bitreplicate(getmsb(a),16), a);
%y = reinterpretcast(y,numerictype(1,32,0));

== matlab function slmips/MIPS/Datapath/RegisterFile/Implementation/ML_impl_noHDL/Write ==
  data: WA3 input fixdt(0,5,0); WD3 input fixdt(0,32,0); WE3 input fixdt(0,1,0); regfile data_store_memory
function fcn(WA3, WD3, WE3)
%#codegen

%Zero based address into one based MATLAB indexing of vectors
global regfile;

if (WE3)
    regfile(WA3+1) = WD3;
end
end

== matlab function slmips/MIPS/Controller/ALUDec/MATLAB Function ==
  data: ALUOp input fixdt(0,2,0); ALUControl output fixdt(0,3,0); funct input fixdt(0,6,0)
function ALUControl = fcn(ALUOp,funct)
%#codegen

ALUControl = fi(0,0,3,0);

switch ALUOp
    case bin2dec('00')
        %add (for lw/sw/addi)
        ALUControl(:) = bin2dec('010');
    case bin2dec('01')
        %sub (for beq)
        ALUControl(:) = bin2dec('110');
    otherwise
        %R-type instructions
        switch funct
            case bin2dec('100000')
                %add
                ALUControl(:) = bin2dec('010');
            case bin2dec('100010')
                %sub
                ALUControl(:) = bin2dec('110');
            case bin2dec('100100')
                %and
                ALUControl(:) = bin2dec('000');
            case bin2dec('100101')
                %or
                ALUControl(:) = bin2dec('001');
            case bin2dec('101010')
                %slt
                ALUControl(:) = bin2dec('111');
            otherwise
                %ILLEGAL OP
                ALUControl(:) = bin2dec('000');
        end
end

== matlab function slmips/MIPS/Controller/MainDec/MATLAB Function ==
  data: op input fixdt(0,6,0); controls output fixdt(0,9,0)
function controls = fcn(op)
%#codegen

controls = fi(0,0,9,0);

switch op
    case bin2dec('000000')
        %RTYPE
        controls(:) = bin2dec('110000010');
    case bin2dec('100011')
        %LW
        controls(:) = bin2dec('101001000');
    case bin2dec('101011')
        %SW
        controls(:) = bin2dec('001010000');
    case bin2dec('000100')
        %BEQ
        controls(:) = bin2dec('000100001');
    case bin2dec('001000')
        %ADDI
        controls(:) = bin2dec('101000000');
    case bin2dec('000010')
        %J
        controls(:) = bin2dec('000000100');
    otherwise
        %ILLEGAL OP
        controls(:) = bin2dec('000000000');
end

== matlab function slmips/Data Memory/MATLAB Function ==
  data: A input fixdt(0,32,0); RD output fixdt(0,32,0); WD input fixdt(0,32,0); WE input fixdt(0,1,0)
function RD = fcn(A, WD, WE)
%#codegen

persistent RAM;
if isempty(RAM)
    %aligned by words
    %64 elements
    RAM = fi(zeros(64, 1), 0, 32, 0);
end

if (WE)
    RAM(bitsliceget(A,8,3)+1) = WD;
end

RD = RAM(bitsliceget(A,8,3)+1);

%disp(RAM(21));

== matlab function slmips/Instruction Memory/MATLAB Function ==
  data: PC input fixdt(0,32,0); Instr output fixdt(0,32,0)
function Instr = fcn(PC)
%#codegen

% mipstest.asm
% David_Harris@hmc.edu, Sarah_Harris@hmc.edu 31 March 2012
% 
% Test the MIPS processor.
% add, sub, and, or, slt, addi, lw, sw, beq, j
% If successful, it should write the value 7 to address 84
%           Assembly            Description             Address    Machine
% main:     addi $2, $0, 5      # initialize $2 = 5     0          20020005
%           addi $3, $0, 12     # initialize $3 = 12    4          2003000c
%           addi $7, $3, -9     # initialize $7 = 3     8          2067fff7
%           or $4, $7, $2       # $4 = (3 OR 5) = 7     c          00e22025
%           and $5, $3, $4      # $5 = (12 AND 7) = 4   10         00642824
%           add $5, $5, $4      # $5 = 4 + 7 = 11       14         00a42820
%           beq $5, $7, end     # shouldn't be taken    18         10a7000a
%           slt $4, $3, $4      # $4 = 12 < 7 = 0       1c         0064202a
%           beq $4, $0, around  # should be taken       20         10800001
%           addi $5, $0, 0      # shouldn't happen      24         20050000
% around:   slt $4, $7, $2      # $4 = 3 < 5 = 1        28         00e2202a
%           add $7, $4, $5      # $7 = 1 + 11 = 12      2c         00853820
%           sub $7, $7, $2      # $7 = 12 - 5 = 7       30         00e23822
%           sw $7, 68($3)       # [80] = 7              34         ac670044
%           lw $2, 80($0)       # $2 = [80] = 7         38         8c020050
%           j end               # should be taken       3c         08000011
%           addi $2, $0, 1      # shouldn't happen      40         20020001
% end:      sw $2, 84($0)       # write mem[84] = 7     44         ac020054

persistent RAM;
if isempty(RAM)
    %aligned by words
    %64 elements
    RAM = fi(zeros(64, 1), 0, 32, 0);
    RAM(1) = hex2dec('20020005');
    RAM(2) = hex2dec('2003000c');
    RAM(3) = hex2dec('2067fff7');
    RAM(4) = hex2dec('00e22025');
    RAM(5) = hex2dec('00642824');
    RAM(6) = hex2dec('00a42820');
    RAM(7) = hex2dec('10a7000a');
    RAM(8) = hex2dec('0064202a');
    RAM(9) = hex2dec('10800001');
    RAM(10) = hex2dec('20050000');
    RAM(11) = hex2dec('00e2202a');
    RAM(12) = hex2dec('00853820');
    RAM(13) = hex2dec('00e23822');
    RAM(14) = hex2dec('ac670044');
    RAM(15) = hex2dec('8c020050');
    %RAM(15) = hex2dec('20020001');
    RAM(16) = hex2dec('08000011');
    RAM(17) = hex2dec('20020001');
    %RAM(16) = hex2dec('8c020050');
    %RAM(17) = hex2dec('08000011');
    RAM(18) = hex2dec('ac020054');
end

%8 because 2^(8-3) = 64 (number of words in RAM)
%3 because PC is aligned by words (4 bytes), therefore two LSB are zeros
Instr = RAM(bitsliceget(PC,8,3)+1);

== matlab function slmips/MIPS/Datapath/RegisterFile/Implementation/ML_impl_noHDL/Read ==
  data: RA1 input fixdt(0,5,0); RD1 output; RA2 input fixdt(0,5,0); RD2 output; regfile data_store_memory
function [RD1, RD2] = fcn(RA1, RA2)
%#codegen

%Zero based address into one based MATLAB indexing of vectors

global regfile;

RD1 = regfile(RA1+1);
RD2 = regfile(RA2+1);
end

== matlab function slmips/MIPS/Datapath/RegisterFile/Implementation/ML_impl/Read ==
  data: RA1 input fixdt(0,5,0); RD1 output; RA2 input fixdt(0,5,0); RD2 output; regfile input
function [RD1, RD2] = fcn(RA1, RA2, regfile)
%#codegen

%Zero based address into one based MATLAB indexing of vectors

RD1 = regfile(RA1+1);
RD2 = regfile(RA2+1);
end

== matlab function slmips/MIPS/Datapath/RegisterFile/Implementation/ML_impl/Write ==
  data: WA3 input fixdt(0,5,0); WD3 input fixdt(0,32,0); WE3 input fixdt(0,1,0); regfile input fixdt(0,32,0); regfile_wr output
function regfile_wr = fcn(WA3, WD3, WE3, regfile)
%#codegen

%Zero based address into one based MATLAB indexing of vectors

regfile_wr = regfile;

if (WE3)
    regfile_wr(WA3+1) = WD3;
end
end
